simulink model "block_model"  (R2020b)
settings: Solver=VariableStepAuto  StartTime=0.0  StopTime=10.0  RelTol=1e-3
model workspace (MAT data in the model file):
  ROBOT_L = 0.145
  ROBOT_T = 0.16
  WHEEL_R = 0.0325
  correction_distance = 0.01
  l_kd = 1
  l_ki = 1
  l_kp = 1
  r_kd = 1
  r_ki = 1
  r_kp = 1
  s_kd = 1
  s_ki = 1
  s_kp = 1
undefined symbols (not defined in the file or in its folder): DiscIntNeverNeededParam
libraries: simulink x8, dspstat3 x3
settings Model: Creator=ped02  LastModifiedBy=ped02

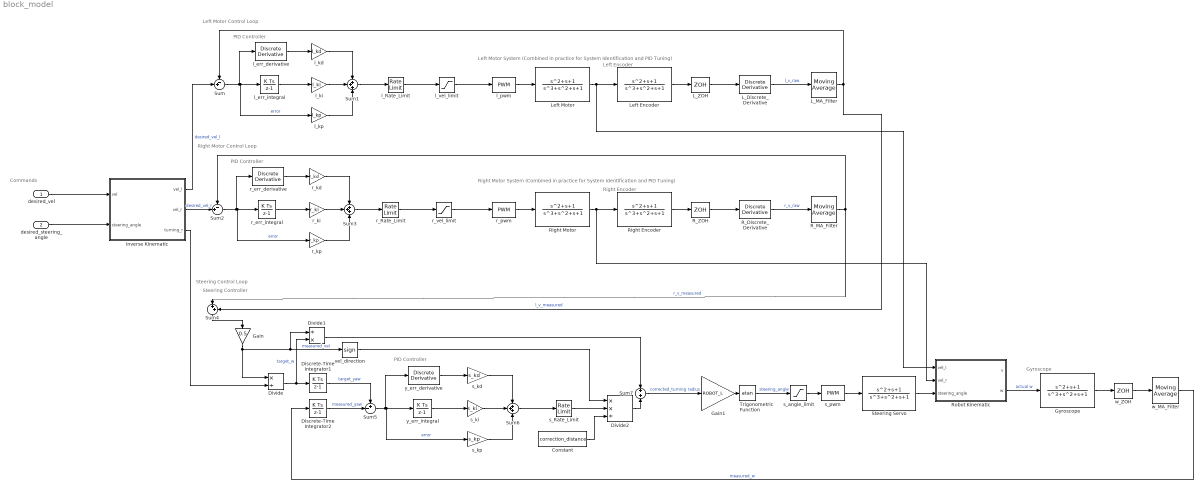
== system block_model ==
  note: Commands
  note: Steering Control Loop
  note: Right Motor Control Loop
  note: Left Motor Control Loop
  note: Gyroscope
  note: Steering Controller
  note: PID Controller
  note: Right Encoder
  note: Left Encoder
  note: PID Controller
  note: PID Controller
  note: Right Motor System (Combined in practice for System Identification and PID Tuning)
  note: Left Motor System (Combined in practice for System Identification and PID Tuning)
  desired_vel : Inport
  desired_steering_angle : Inport  Port=2
  Constant : Constant  Value=correction_distance
  Discrete-Time Integrator1 : DiscreteIntegrator  SampleTime=-1  ICPrevOutput=DiscIntNeverNeededParam  ICPrevScaledInput=DiscIntNeverNeededParam
  Discrete-Time Integrator2 : DiscreteIntegrator  SampleTime=-1  ICPrevOutput=DiscIntNeverNeededParam  ICPrevScaledInput=DiscIntNeverNeededParam
  Divide : Product  Inputs=*/
  Divide1 : Product  Inputs=/*
  Divide2 : Product  Inputs=**/
  Gain : Gain  Gain=0.5
  Gain1 : Gain  Gain=ROBOT_L
  Gyroscope : TransferFcn  Numerator=[1 1 1]  Denominator=[1 1 1 1]
  Inverse Kinematic : Subsystem  mask{ROBOT_T=ROBOT_T, ROBOT_L=ROBOT_L, WHEEL_R=WHEEL_R}
  L_Discrete_Derivative : simulink/Discrete/Discrete Derivative  gainval=1.0  ICPrevScaledInput=0.0  OutMin=[]  OutMax=[]  OutDataType=fixdt(1, 16)  OutScaling=2^-10  DoSatur=off
  L_MA_Filter : dspstat3/Moving Average  Method=Sliding window  ForgettingFactorPort=off  SpecifyWindowLength=on  WindowLength=4  ForgettingFactor=0.9  SimulateUsing=Code generation
  L_ZOH : ZeroOrderHold  SampleTime=-1
  Left Encoder : TransferFcn  Numerator=[1 1 1]  Denominator=[1 1 1 1]
  Left Motor : TransferFcn  Numerator=[1 1 1]  Denominator=[1 1 1 1]
  R_Discrete_Derivative : simulink/Discrete/Discrete Derivative  gainval=1.0  ICPrevScaledInput=0.0  OutMin=[]  OutMax=[]  OutDataType=fixdt(1, 16)  OutScaling=2^-10  DoSatur=off
  R_MA_Filter : dspstat3/Moving Average  Method=Sliding window  ForgettingFactorPort=off  SpecifyWindowLength=on  WindowLength=4  ForgettingFactor=0.9  SimulateUsing=Code generation
  R_ZOH : ZeroOrderHold  SampleTime=-1
  Right Encoder : TransferFcn  Numerator=[1 1 1]  Denominator=[1 1 1 1]
  Right Motor : TransferFcn  Numerator=[1 1 1]  Denominator=[1 1 1 1]
  Robot Kinematic : Subsystem
  Steering Servo : TransferFcn  Numerator=[1 1 1]  Denominator=[1 1 1 1]
  Sum : Sum  Inputs=-+|
  Sum1 : Sum  Inputs=+++
  Sum2 : Sum  Inputs=-+|
  Sum3 : Sum  Inputs=+++
  Sum4 : Sum  Inputs=|++
  Sum5 : Sum  Inputs=+-|
  Sum6 : Sum  Inputs=+++
  Sum7 : Sum  Inputs=+|+
  Trigonometric Function : Trigonometry  Operator=atan
  l_Rate_Limit : RateLimiter  SampleTimeMode=inherited
  l_err_derivative : simulink/Discrete/Discrete Derivative  gainval=1.0  ICPrevScaledInput=0.0  OutMin=[]  OutMax=[]  OutDataType=fixdt(1, 16)  OutScaling=2^-10  DoSatur=off
  l_err_integral : DiscreteIntegrator  SampleTime=-1  ICPrevOutput=DiscIntNeverNeededParam  ICPrevScaledInput=DiscIntNeverNeededParam
  l_kd : Gain  Gain=l_kd
  l_ki : Gain  Gain=l_ki
  l_kp : Gain  Gain=l_kp
  l_pwm : simulink/Discontinuities/PWM  DisableCoverage=on  Period=1  DisallowZeroDutyCycle=off  RunAtFixedTimeIntervals=off  SampleTime=0.1
  l_vel_limit : Saturate
  r_Rate_Limit : RateLimiter  SampleTimeMode=inherited
  r_err_derivative : simulink/Discrete/Discrete Derivative  gainval=1.0  ICPrevScaledInput=0.0  OutMin=[]  OutMax=[]  OutDataType=fixdt(1, 16)  OutScaling=2^-10  DoSatur=off
  r_err_integral : DiscreteIntegrator  SampleTime=-1  ICPrevOutput=DiscIntNeverNeededParam  ICPrevScaledInput=DiscIntNeverNeededParam
  r_kd : Gain  Gain=r_kd
  r_ki : Gain  Gain=r_ki
  r_kp : Gain  Gain=r_kp
  r_pwm : simulink/Discontinuities/PWM  DisableCoverage=on  Period=1  DisallowZeroDutyCycle=off  RunAtFixedTimeIntervals=off  SampleTime=0.1
  r_vel_limit : Saturate
  s_Rate_Limit : RateLimiter  SampleTimeMode=inherited
  s_angle_limit : Saturate
  s_kd : Gain  Gain=s_kd
  s_ki : Gain  Gain=s_ki
  s_kp : Gain  Gain=s_kp
  s_pwm : simulink/Discontinuities/PWM  DisableCoverage=on  Period=1  DisallowZeroDutyCycle=off  RunAtFixedTimeIntervals=off  SampleTime=0.1
  vel_direction : Signum
  w_MA_Filter : dspstat3/Moving Average  Method=Sliding window  ForgettingFactorPort=off  SpecifyWindowLength=on  WindowLength=4  ForgettingFactor=0.9  SimulateUsing=Code generation
  w_ZOH : ZeroOrderHold  SampleTime=-1
  y_err_derivative : simulink/Discrete/Discrete Derivative  gainval=1.0  ICPrevScaledInput=0.0  OutMin=[]  OutMax=[]  OutDataType=fixdt(1, 16)  OutScaling=2^-10  DoSatur=off
  y_err_integral : DiscreteIntegrator  SampleTime=-1  ICPrevOutput=DiscIntNeverNeededParam  ICPrevScaledInput=DiscIntNeverNeededParam
  wires:
  Sum7/1 -> Gain1/1  "corrected_turning radius"
  Steering Servo/1 -> Robot Kinematic/3(steering_angle)
  s_Rate_Limit/1 -> Divide2/2
  s_pwm/1 -> Steering Servo/1
  desired_steering_angle/1 -> Inverse Kinematic/2(steering_angle)
  desired_vel/1 -> Inverse Kinematic/1(vel)
  r_err_integral/1 -> r_ki/1
  Sum2/1 -> r_err_integral/1, r_kp/1, r_err_derivative/1  "error"
  r_Rate_Limit/1 -> r_vel_limit/1
  Trigonometric Function/1 -> s_angle_limit/1  "steering_angle"
  Gain1/1 -> Trigonometric Function/1
  Discrete-Time Integrator1/1 -> Sum5/1  "target_yaw"
  Divide2/1 -> Sum7/2
  Divide1/1 -> Sum7/1
  Divide/1 -> Discrete-Time Integrator1/1, Divide1/2  "target_w"
  Constant/1 -> Divide2/3
  vel_direction/1 -> Divide2/1
  l_err_integral/1 -> l_ki/1
  Discrete-Time Integrator2/1 -> Sum5/2  "measured_yaw"
  Sum4/1 -> Gain/1
  Sum5/1 -> s_kp/1, y_err_integral/1, y_err_derivative/1  "error"
  Gain/1 -> Divide/1, vel_direction/1, Divide1/1  "measured_vel"
  s_kd/1 -> Sum6/1
  Right Encoder/1 -> R_ZOH/1
  r_kd/1 -> Sum3/1
  r_ki/1 -> Sum3/2
  r_kp/1 -> Sum3/3
  w_ZOH/1 -> w_MA_Filter/1
  s_ki/1 -> Sum6/2
  Right Motor/1 -> Right Encoder/1, Robot Kinematic/2(vel_r)
  y_err_derivative/1 -> s_kd/1
  s_kp/1 -> Sum6/3
  y_err_integral/1 -> s_ki/1
  Gyroscope/1 -> w_ZOH/1
  l_Rate_Limit/1 -> l_vel_limit/1
  Left Motor/1 -> Left Encoder/1, Robot Kinematic/1(vel_l)
  Sum/1 -> l_kp/1, l_err_integral/1, l_err_derivative/1  "error"
  L_Discrete_Derivative/1 -> L_MA_Filter/1  "l_v_raw"
  l_pwm/1 -> Left Motor/1
  L_MA_Filter/1 -> Sum/1, Sum4/2  "l_v_measured"
  Left Encoder/1 -> L_ZOH/1
  l_err_derivative/1 -> l_kd/1
  l_kd/1 -> Sum1/1
  l_ki/1 -> Sum1/2
  l_kp/1 -> Sum1/3
  r_pwm/1 -> Right Motor/1
  r_err_derivative/1 -> r_kd/1
  R_Discrete_Derivative/1 -> R_MA_Filter/1  "r_v_raw"
  R_MA_Filter/1 -> Sum2/1, Sum4/1  "r_v_measured"
  Inverse Kinematic/2(vel_r) -> Sum2/2  "desired_vel_r"
  Inverse Kinematic/1(vel_l) -> Sum/2  "desired_vel_l"
  Robot Kinematic/2(w) -> Gyroscope/1  "actual w"
  Inverse Kinematic/3(turning_r) -> Divide/2
  Sum3/1 -> r_Rate_Limit/1
  s_angle_limit/1 -> s_pwm/1
  w_MA_Filter/1 -> Discrete-Time Integrator2/1  "measured_w"
  Sum6/1 -> s_Rate_Limit/1
  Sum1/1 -> l_Rate_Limit/1
  l_vel_limit/1 -> l_pwm/1
  r_vel_limit/1 -> r_pwm/1
  L_ZOH/1 -> L_Discrete_Derivative/1
  R_ZOH/1 -> R_Discrete_Derivative/1

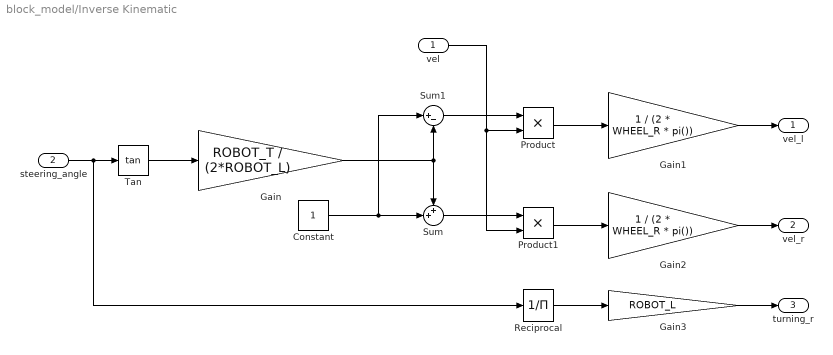
== system block_model/Inverse Kinematic ==
  vel : Inport
  steering_angle : Inport  Port=2
  Constant : Constant
  Gain : Gain  Gain=ROBOT_T / (2*ROBOT_L)
  Gain1 : Gain  Gain=1 / (2 * WHEEL_R * pi())
  Gain2 : Gain  Gain=1 / (2 * WHEEL_R * pi())
  Gain3 : Gain  Gain=ROBOT_L
  Product : Product
  Product1 : Product
  Reciprocal : Product  Inputs=/
  Sum : Sum  Inputs=++|
  Sum1 : Sum  Inputs=|+-
  Tan : Trigonometry  Operator=tan
  vel_l : Outport
  vel_r : Outport  Port=2
  turning_r : Outport  Port=3
  wires:
  steering_angle/1 -> Reciprocal/1, Tan/1
  Tan/1 -> Gain/1
  Constant/1 -> Sum1/1, Sum/2
  Gain/1 -> Sum/1, Sum1/2
  Sum1/1 -> Product/1
  vel/1 -> Product1/2, Product/2
  Sum/1 -> Product1/1
  Product1/1 -> Gain2/1
  Product/1 -> Gain1/1
  Gain1/1 -> vel_l/1
  Gain2/1 -> vel_r/1
  Reciprocal/1 -> Gain3/1
  Gain3/1 -> turning_r/1

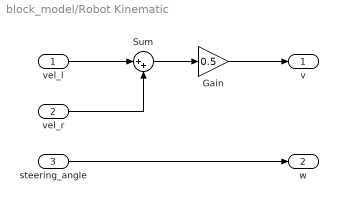
== system block_model/Robot Kinematic ==
  vel_l : Inport
  vel_r : Inport  Port=2
  steering_angle : Inport  Port=3
  Gain : Gain  Gain=0.5
  Sum : Sum  Inputs=|++
  v : Outport
  w : Outport  Port=2
  wires:
  steering_angle/1 -> w/1
  vel_l/1 -> Sum/1
  vel_r/1 -> Sum/2
  Sum/1 -> Gain/1
  Gain/1 -> v/1
